simulink model "krzywdalab8_tf_si"  (R2023b)
settings: Solver=VariableStepAuto  StartTime=0.0  StopTime=10.0  RelTol=1e-3
values from neighbouring files (symbols this model uses):
  flow_input_step_1 = 0.1 * flow_input_max_1    [feedback_cascade_state.m]    (also in feedback_cascade_transfer_function.m)
  flow_input_step_2 = 0    [feedback_cascade_state.m]    (also in feedback_cascade_transfer_function.m)
  initial_height_1 = flow_inputs_vec_1(i) / a_1 + initial_height_2    [feedback_cascade_state.m]    (also in feedback_cascade_transfer_function.m)
  initial_height_2 = (flow_input_max_2 + initial_flow_input_1) / a_2    [feedback_cascade_state.m]    (also in feedback_cascade_transfer_function.m)
  M = [(A1 * A2) (a_1 * A1 + a_2 * A1 + a_1 * A2) a_1*a_2]    [feedback_cascade_transfer_function.m]    (also in krzywdalab8.m = [(A1*A2) (a1*A1+a2*A1+a1*A2) a1*a2])
  N_11 = [A2 (a_1 + a_2)]    [feedback_cascade_transfer_function.m]    (also in krzywdalab8.m = [A2 (a1+a2)])
  N_21 = [a_1]    [feedback_cascade_transfer_function.m]    (also in krzywdalab8.m = [a1])
  N_22 = [A1 a_1]    [feedback_cascade_transfer_function.m]    (also in krzywdalab8.m = [A1 a1])
  T0 = 2    [feedback_cascade_state.m]    (also in feedback_cascade_transfer_function.m; krzywdalab8.m)
settings Model: Creator=igorkrzywda  LastModifiedBy=igorkrzywda

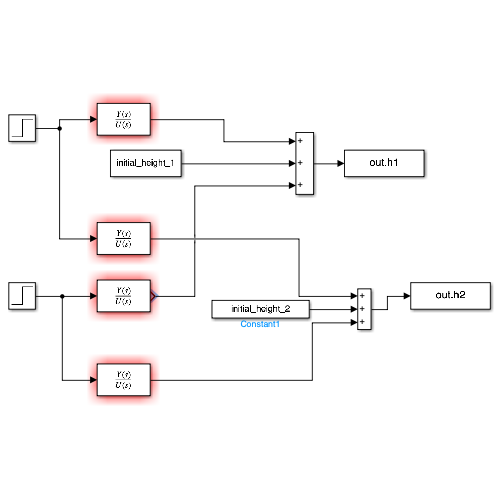
[thumbnail: Simulink's stored preview of the top-level diagram]
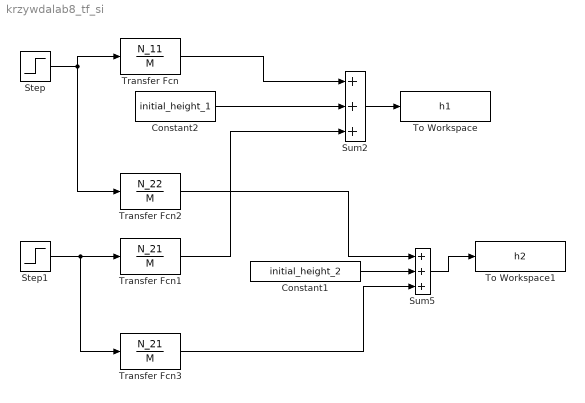
== system krzywdalab8_tf_si ==
  Constant1 : Constant  Value=initial_height_2
  Constant2 : Constant  Value=initial_height_1
  Step : Step  Time=T0  After=flow_input_step_1  SampleTime=0
  Step1 : Step  Time=T0  After=flow_input_step_2  SampleTime=0
  Sum2 : Sum  Inputs=+++
  Sum5 : Sum  Inputs=+++
  To Workspace : ToWorkspace  VariableName=h1  SampleTime=-1
  To Workspace1 : ToWorkspace  VariableName=h2  SampleTime=-1
  Transfer Fcn : TransferFcn  Numerator=N_11  Denominator=M
  Transfer Fcn1 : TransferFcn  Numerator=N_21  Denominator=M
  Transfer Fcn2 : TransferFcn  Numerator=N_22  Denominator=M
  Transfer Fcn3 : TransferFcn  Numerator=N_21  Denominator=M
  wires:
  Step/1 -> Transfer Fcn2/1, Transfer Fcn/1
  Step1/1 -> Transfer Fcn3/1, Transfer Fcn1/1
  Transfer Fcn1/1 -> Sum2/3
  Constant1/1 -> Sum5/2
  Transfer Fcn/1 -> Sum2/1
  Sum2/1 -> To Workspace/1
  Transfer Fcn3/1 -> Sum5/3
  Sum5/1 -> To Workspace1/1
  Transfer Fcn2/1 -> Sum5/1
  Constant2/1 -> Sum2/2
